simulink model "final_version"  (R2024b)
settings: Solver=FixedStepAuto  StartTime=0.0  StopTime=inf  RelTol=1e-3  EnableMultiTasking=on
libraries: simulink x46, stm32f4xxblockslib x20, dspstat3 x2, stm32blockslib x1
(part 2 of 2)

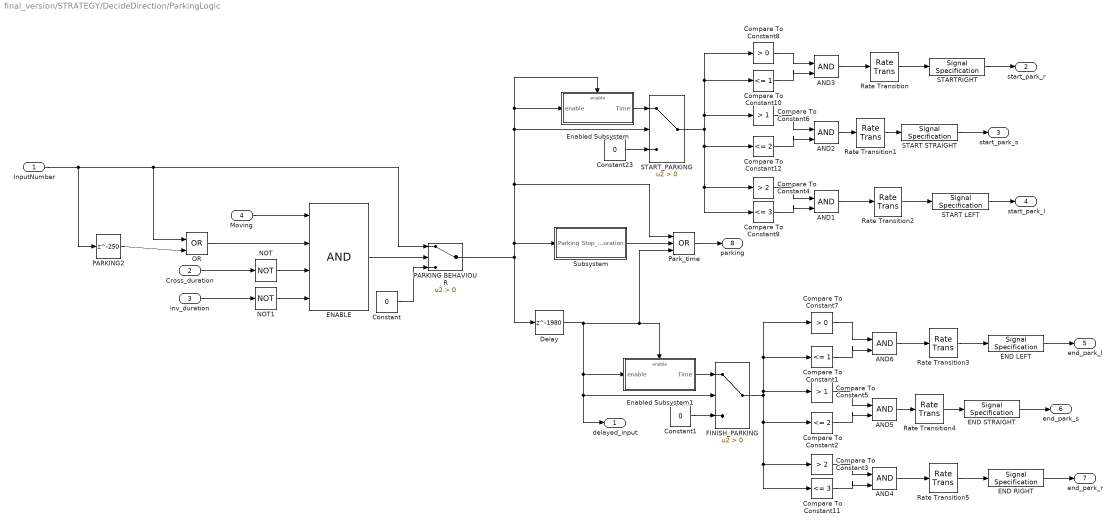
== system final_version/STRATEGY/DecideDirection/ParkingLogic ==
  InputNumber : Inport
  Cross_duration : Inport  Port=2
  inv_duration : Inport  Port=3
  Moving : Inport  Port=4
  AND{1..6} (6 alike) : Logic  IconShape=distinctive  AllPortsSameDT=off  OutDataTypeStr=boolean
  Compare To Constant1 : simulink/Logic and Bit Operations/Compare To Constant  relop=<=  const=1  OutDataTypeStr=boolean
  Compare To Constant10 : simulink/Logic and Bit Operations/Compare To Constant  relop=<=  const=1  OutDataTypeStr=boolean
  Compare To Constant11 : simulink/Logic and Bit Operations/Compare To Constant  relop=<=  const=3  OutDataTypeStr=boolean
  Compare To Constant12 : simulink/Logic and Bit Operations/Compare To Constant  relop=<=  const=2  OutDataTypeStr=boolean
  Compare To Constant2 : simulink/Logic and Bit Operations/Compare To Constant  relop=<=  const=2  OutDataTypeStr=boolean
  Compare To Constant3 : simulink/Logic and Bit Operations/Compare To Constant  relop=>  const=2  OutDataTypeStr=boolean
  Compare To Constant4 : simulink/Logic and Bit Operations/Compare To Constant  relop=>  const=2  OutDataTypeStr=boolean
  Compare To Constant5 : simulink/Logic and Bit Operations/Compare To Constant  relop=>  const=1  OutDataTypeStr=boolean
  Compare To Constant6 : simulink/Logic and Bit Operations/Compare To Constant  relop=>  const=1  OutDataTypeStr=boolean
  Compare To Constant7 : simulink/Logic and Bit Operations/Compare To Constant  relop=>  const=0  OutDataTypeStr=boolean
  Compare To Constant8 : simulink/Logic and Bit Operations/Compare To Constant  relop=>  const=0  OutDataTypeStr=boolean
  Compare To Constant9 : simulink/Logic and Bit Operations/Compare To Constant  relop=<=  const=3  OutDataTypeStr=boolean
  Constant : Constant  Value=0
  Constant1 : Constant  Value=0
  Constant23 : Constant  Value=0
  Delay : Delay  DelayLength=1980
  ENABLE : Logic  Inputs=4  IconShape=distinctive  AllPortsSameDT=off  OutDataTypeStr=boolean
  END LEFT : SignalSpecification
  END RIGHT : SignalSpecification
  END STRAIGHT : SignalSpecification
  Enabled Subsystem : Subsystem  TreatAsAtomicUnit=on
  Enabled Subsystem1 : Subsystem  TreatAsAtomicUnit=on
  FINISH_PARKING : Switch  Criteria=u2 > Threshold  SaturateOnIntegerOverflow=off  InputSameDT=off
  NOT : Logic  Operator=NOT  IconShape=distinctive  AllPortsSameDT=off  OutDataTypeStr=boolean
  NOT1 : Logic  Operator=NOT  IconShape=distinctive  AllPortsSameDT=off  OutDataTypeStr=boolean
  OR : Logic  Operator=OR  IconShape=distinctive  AllPortsSameDT=off  OutDataTypeStr=boolean
  PARKING BEHAVIOUR : Switch  Criteria=u2 > Threshold  SaturateOnIntegerOverflow=off  InputSameDT=off
  PARKING2 : Delay  DelayLength=250
  Park_time : Logic  Operator=OR  Inputs=3  IconShape=distinctive  AllPortsSameDT=off  OutDataTypeStr=boolean
  Rate Transition{,1..5} (6 alike) : RateTransition
  START LEFT : SignalSpecification
  START STRAIGHT : SignalSpecification
  STARTRIGHT : SignalSpecification
  START_PARKING : Switch  Criteria=u2 > Threshold  SaturateOnIntegerOverflow=off  InputSameDT=off
  Subsystem : Subsystem
  delayed_input : Outport
  start_park_r : Outport  Port=2
  start_park_s : Outport  Port=3
  "start_park_l " : Outport  Port=4
  end_park_l : Outport  Port=5
  end_park_s : Outport  Port=6
  end_park_r : Outport  Port=7
  parking : Outport  Port=8
  wires:
  InputNumber/1 -> PARKING BEHAVIOUR/1, OR/1, PARKING2/1
  FINISH_PARKING/1 -> Compare To Constant1/1, Compare To Constant7/1, Compare To Constant5/1, Compare To Constant2/1, Compare To Constant3/1, Compare To Constant11/1
  START_PARKING/1 -> Compare To Constant8/1, Compare To Constant10/1, Compare To Constant6/1, Compare To Constant12/1, Compare To Constant4/1, Compare To Constant9/1
  PARKING BEHAVIOUR/1 -> Delay/1, Subsystem/1(Parking), Park_time/1, START_PARKING/2, Enabled Subsystem/1(enable), Enabled Subsystem/Enable
  NOT1/1 -> ENABLE/4
  inv_duration/1 -> NOT1/1
  PARKING2/1 -> OR/2
  OR/1 -> ENABLE/2
  Moving/1 -> ENABLE/1
  NOT/1 -> ENABLE/3
  Cross_duration/1 -> NOT/1
  ENABLE/1 -> PARKING BEHAVIOUR/2
  Constant/1 -> PARKING BEHAVIOUR/3
  Compare To Constant8/1 -> AND3/1
  Compare To Constant10/1 -> AND3/2
  Compare To Constant6/1 -> AND2/1
  Compare To Constant12/1 -> AND2/2
  Compare To Constant4/1 -> AND1/1
  Compare To Constant9/1 -> AND1/2
  AND1/1 -> Rate Transition2/1
  Rate Transition2/1 -> START LEFT/1
  START LEFT/1 -> "start_park_l "/1
  START STRAIGHT/1 -> start_park_s/1
  STARTRIGHT/1 -> start_park_r/1
  Rate Transition/1 -> STARTRIGHT/1
  Rate Transition1/1 -> START STRAIGHT/1
  AND2/1 -> Rate Transition1/1
  AND3/1 -> Rate Transition/1
  Constant23/1 -> START_PARKING/3
  Enabled Subsystem/1(Time) -> START_PARKING/1
  Delay/1 -> Park_time/3, Enabled Subsystem1/Enable, Enabled Subsystem1/1(enable), delayed_input/1, FINISH_PARKING/2
  Park_time/1 -> parking/1
  Subsystem/1(Stop_duration) -> Park_time/2
  Constant1/1 -> FINISH_PARKING/3
  Enabled Subsystem1/1(Time) -> FINISH_PARKING/1
  Compare To Constant1/1 -> AND6/2
  Compare To Constant7/1 -> AND6/1
  Compare To Constant5/1 -> AND5/1
  Compare To Constant2/1 -> AND5/2
  Compare To Constant3/1 -> AND4/1
  Compare To Constant11/1 -> AND4/2
  AND4/1 -> Rate Transition5/1
  Rate Transition5/1 -> END RIGHT/1
  END RIGHT/1 -> end_park_r/1
  END STRAIGHT/1 -> end_park_s/1
  END LEFT/1 -> end_park_l/1
  Rate Transition3/1 -> END LEFT/1
  Rate Transition4/1 -> END STRAIGHT/1
  AND5/1 -> Rate Transition4/1
  AND6/1 -> Rate Transition3/1

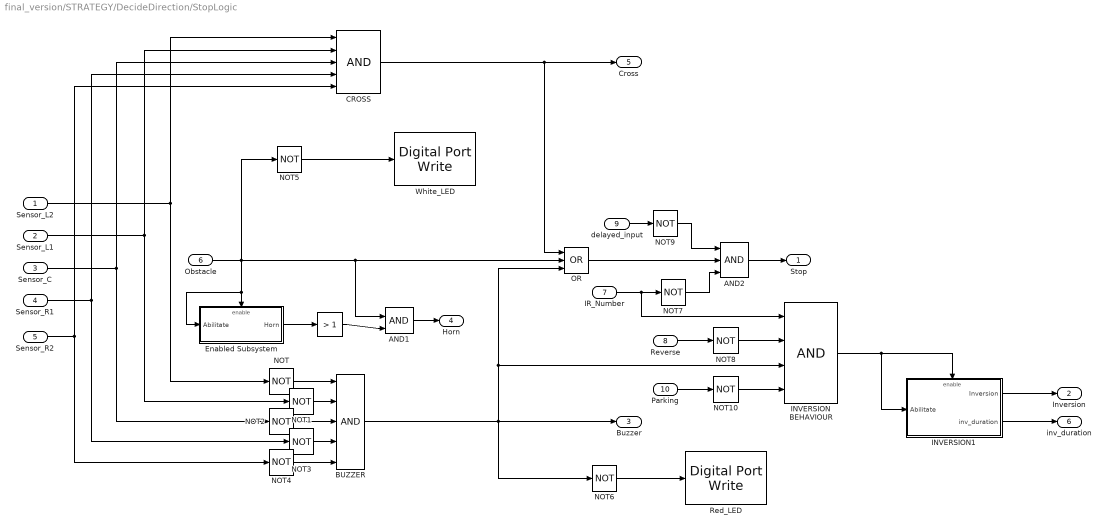
== system final_version/STRATEGY/DecideDirection/StopLogic ==
  Sensor_L2 : Inport
  Sensor_L1 : Inport  Port=2
  Sensor_C : Inport  Port=3
  Sensor_R1 : Inport  Port=4
  Sensor_R2 : Inport  Port=5
  Obstacle : Inport  Port=6
  IR_Number : Inport  Port=7
  Reverse : Inport  Port=8
  delayed_input : Inport  Port=9
  Parking : Inport  Port=10
  " " : simulink/Logic and Bit Operations/Compare To Constant  relop=>  const=1  OutDataTypeStr=boolean
  AND1 : Logic  IconShape=distinctive  AllPortsSameDT=off  OutDataTypeStr=boolean
  AND2 : Logic  Inputs=3  IconShape=distinctive  AllPortsSameDT=off  OutDataTypeStr=boolean
  BUZZER : Logic  Inputs=5  IconShape=distinctive  AllPortsSameDT=off  OutDataTypeStr=boolean
  CROSS : Logic  Inputs=5  IconShape=distinctive  AllPortsSameDT=off  OutDataTypeStr=boolean
  Enabled Subsystem : Subsystem  TreatAsAtomicUnit=on
  INVERSION BEHAVIOUR : Logic  Inputs=4  IconShape=distinctive  AllPortsSameDT=off  OutDataTypeStr=boolean
  INVERSION1 : Subsystem  TreatAsAtomicUnit=on
  NOT{,1..10} (11 alike) : Logic  Operator=NOT  IconShape=distinctive  AllPortsSameDT=off  OutDataTypeStr=boolean
  OR : Logic  Operator=OR  Inputs=3  IconShape=distinctive  AllPortsSameDT=off  OutDataTypeStr=boolean
  Red_LED : stm32f4xxblockslib/Digital Port Write  PortName=GPIOC  PinNumber=[6]  ReadOperation=off  IOAsArray=on  EnableSimPort=off  hoistedMaskSrc=ECSoC/ECSimCodegen/Digital Port Write
  White_LED : stm32f4xxblockslib/Digital Port Write  PortName=GPIOC  PinNumber=[9]  ReadOperation=off  IOAsArray=on  EnableSimPort=off  hoistedMaskSrc=ECSoC/ECSimCodegen/Digital Port Write
  Stop : Outport
  Inversion : Outport  Port=2
  Buzzer : Outport  Port=3
  Horn : Outport  Port=4
  Cross : Outport  Port=5
  inv_duration : Outport  Port=6
  wires:
  Sensor_L2/1 -> NOT/1, CROSS/1
  Sensor_L1/1 -> CROSS/2, NOT1/1
  Sensor_C/1 -> CROSS/3, NOT2/1
  Sensor_R1/1 -> CROSS/4, NOT3/1
  Sensor_R2/1 -> CROSS/5, NOT4/1
  CROSS/1 -> Cross/1, OR/1
  NOT/1 -> BUZZER/1
  NOT1/1 -> BUZZER/2
  NOT2/1 -> BUZZER/3
  NOT3/1 -> BUZZER/4
  NOT4/1 -> BUZZER/5
  Obstacle/1 -> NOT5/1, AND1/1, OR/2, Enabled Subsystem/1(Abilitate), Enabled Subsystem/Enable
  Enabled Subsystem/1(Horn) -> " "/1
  NOT5/1 -> White_LED/1
  NOT6/1 -> Red_LED/1
  INVERSION1/1(Inversion) -> Inversion/1
  AND2/1 -> Stop/1
  IR_Number/1 -> NOT7/1, INVERSION BEHAVIOUR/1
  AND1/1 -> Horn/1
  " "/1 -> AND1/2
  Reverse/1 -> NOT8/1
  BUZZER/1 -> NOT6/1, OR/3, INVERSION BEHAVIOUR/3, Buzzer/1
  NOT7/1 -> AND2/3
  OR/1 -> AND2/2
  delayed_input/1 -> NOT9/1
  NOT9/1 -> AND2/1
  NOT8/1 -> INVERSION BEHAVIOUR/2
  Parking/1 -> NOT10/1
  NOT10/1 -> INVERSION BEHAVIOUR/4
  INVERSION BEHAVIOUR/1 -> INVERSION1/1(Abilitate), INVERSION1/Enable
  INVERSION1/2(inv_duration) -> inv_duration/1

== system final_version/STRATEGY/DecideDirection/TurnLeftLogic ==
  Sensor_L2 : Inport
  Sensor_L1 : Inport  Port=2
  Sensor_C : Inport  Port=3
  Inversion : Inport  Port=4
  cross_duration : Inport  Port=5
  start_park_r : Inport  Port=6
  end_park_r : Inport  Port=7
  AND : Logic  IconShape=distinctive  AllPortsSameDT=off  OutDataTypeStr=boolean
  AND1 : Logic  Inputs=3  IconShape=distinctive  AllPortsSameDT=off  OutDataTypeStr=boolean
  AND2 : Logic  Inputs=5  IconShape=distinctive  AllPortsSameDT=off  OutDataTypeStr=boolean
  NOT{1..5} (5 alike) : Logic  Operator=NOT  IconShape=distinctive  AllPortsSameDT=off  OutDataTypeStr=boolean
  OR : Logic  Operator=OR  IconShape=distinctive  AllPortsSameDT=off  OutDataTypeStr=boolean
  Turn_Left : Outport
  wires:
  NOT3/1 -> AND/2
  AND/1 -> OR/1
  Sensor_L1/1 -> NOT3/1, AND1/1
  Sensor_L2/1 -> AND1/2, AND/1
  Sensor_C/1 -> AND1/3
  AND1/1 -> OR/2
  Inversion/1 -> NOT1/1
  OR/1 -> AND2/1
  NOT1/1 -> AND2/2
  AND2/1 -> Turn_Left/1
  NOT2/1 -> AND2/3
  cross_duration/1 -> NOT2/1
  start_park_r/1 -> NOT4/1
  NOT4/1 -> AND2/4
  end_park_r/1 -> NOT5/1
  NOT5/1 -> AND2/5

== system final_version/STRATEGY/DecideDirection/TurnRightLogic ==
  Sensor_R2 : Inport
  Sensor_R1 : Inport  Port=2
  Sensor_C : Inport  Port=3
  inversion : Inport  Port=4
  cross_duration : Inport  Port=5
  start_park_r : Inport  Port=6
  end_park_r : Inport  Port=7
  AND : Logic  Inputs=3  IconShape=distinctive  AllPortsSameDT=off  OutDataTypeStr=boolean
  AND1 : Logic  IconShape=distinctive  AllPortsSameDT=off  OutDataTypeStr=boolean
  AND2 : Logic  Inputs=4  IconShape=distinctive  AllPortsSameDT=off  OutDataTypeStr=boolean
  NOT{1..4} (4 alike) : Logic  Operator=NOT  IconShape=distinctive  AllPortsSameDT=off  OutDataTypeStr=boolean
  OR1 : Logic  Operator=OR  IconShape=distinctive  AllPortsSameDT=off  OutDataTypeStr=boolean
  XOR : Logic  Operator=XOR  IconShape=distinctive  AllPortsSameDT=off  OutDataTypeStr=boolean
  Turn_Right : Outport
  wires:
  AND1/1 -> OR1/1
  NOT4/1 -> AND1/2
  Sensor_R1/1 -> AND/1, NOT4/1
  Sensor_R2/1 -> AND/2, AND1/1
  inversion/1 -> XOR/2
  AND/1 -> OR1/2
  Sensor_C/1 -> AND/3
  AND2/1 -> Turn_Right/1
  NOT1/1 -> AND2/2
  cross_duration/1 -> NOT1/1
  start_park_r/1 -> NOT2/1
  NOT2/1 -> AND2/3
  end_park_r/1 -> NOT3/1
  NOT3/1 -> AND2/4
  XOR/1 -> AND2/1
  OR1/1 -> XOR/1

== system final_version/STRATEGY/DecideDirection/TurnSlightLeftLogic ==
  Sensor_C : Inport
  Sensor_L1 : Inport  Port=2
  Sensor_L2 : Inport  Port=3
  start_park_l : Inport  Port=4
  end_park_l : Inport  Port=5
  start_park_r : Inport  Port=6
  end_park_r : Inport  Port=7
  Inversion : Inport  Port=8
  x_left : Inport  Port=9
  AND : Logic  Inputs=3  IconShape=distinctive  AllPortsSameDT=off  OutDataTypeStr=boolean
  AND1 : Logic  Inputs=4  IconShape=distinctive  AllPortsSameDT=off  OutDataTypeStr=boolean
  NOT{,1..3} (4 alike) : Logic  Operator=NOT  IconShape=distinctive  AllPortsSameDT=off  OutDataTypeStr=boolean
  OR : Logic  Operator=OR  Inputs=4  IconShape=distinctive  AllPortsSameDT=off  OutDataTypeStr=boolean
  TurnSlightLeft : Outport
  wires:
  Sensor_C/1 -> NOT/1
  Sensor_L1/1 -> AND/2
  NOT/1 -> AND/1
  AND/1 -> OR/1
  end_park_l/1 -> OR/3
  AND1/1 -> TurnSlightLeft/1
  OR/1 -> AND1/1
  NOT1/1 -> AND1/2
  start_park_r/1 -> NOT1/1
  start_park_l/1 -> OR/2
  Sensor_L2/1 -> AND/3
  Inversion/1 -> NOT2/1
  NOT2/1 -> AND1/3
  x_left/1 -> OR/4
  end_park_r/1 -> NOT3/1
  NOT3/1 -> AND1/4

== system final_version/STRATEGY/DecideDirection/TurnSlightRightLogic ==
  Sensor_R1 : Inport
  Sensor_R2 : Inport  Port=2
  Sensor_C : Inport  Port=3
  start_park_r : Inport  Port=4
  end_park_r : Inport  Port=5
  Inversion : Inport  Port=6
  x_right : Inport  Port=7
  AND : Logic  Inputs=3  IconShape=distinctive  AllPortsSameDT=off  OutDataTypeStr=boolean
  AND1 : Logic  IconShape=distinctive  AllPortsSameDT=off  OutDataTypeStr=boolean
  NOT1 : Logic  Operator=NOT  IconShape=distinctive  AllPortsSameDT=off  OutDataTypeStr=boolean
  NOT2 : Logic  Operator=NOT  IconShape=distinctive  AllPortsSameDT=off  OutDataTypeStr=boolean
  OR : Logic  Operator=OR  Inputs=4  IconShape=distinctive  AllPortsSameDT=off  OutDataTypeStr=boolean
  TurnSlightRight : Outport
  wires:
  Sensor_C/1 -> NOT2/1
  Sensor_R1/1 -> AND/1
  AND/1 -> OR/1
  end_park_r/1 -> OR/3
  start_park_r/1 -> OR/2
  NOT2/1 -> AND/3
  Sensor_R2/1 -> AND/2
  AND1/1 -> TurnSlightRight/1
  OR/1 -> AND1/1
  Inversion/1 -> NOT1/1
  NOT1/1 -> AND1/2
  x_right/1 -> OR/4

== system final_version/STRATEGY/DecideDirection/UltrasonicLogic ==
  UT : Inport
  Clock : Clock
  Clock1 : Clock
  Constant : Constant  Value=11.7
  Constant1 : Constant  Value=9.3
  OBSTACLE : RelationalOperator  Operator=<  OutDataTypeStr=boolean  RndMeth=Simplest  InputSameDT=off
  REVERSE : RelationalOperator  Operator=<  OutDataTypeStr=boolean  RndMeth=Simplest  InputSameDT=off
  obstacle : Logic  IconShape=distinctive  AllPortsSameDT=off  OutDataTypeStr=boolean
  obstacle clock : simulink/Logic and Bit Operations/Compare To Constant  relop=>=  const=0.25  OutDataTypeStr=boolean
  reverse : Logic  IconShape=distinctive  AllPortsSameDT=off  OutDataTypeStr=boolean
  reverse clock : simulink/Logic and Bit Operations/Compare To Constant  relop=>=  const=0.25  OutDataTypeStr=boolean
  Obstacle : Outport
  Reverse : Outport  Port=2
  wires:
  Clock1/1 -> reverse clock/1
  Constant1/1 -> REVERSE/2
  Clock/1 -> obstacle clock/1
  reverse clock/1 -> reverse/2
  Constant/1 -> OBSTACLE/2
  UT/1 -> OBSTACLE/1, REVERSE/1
  obstacle clock/1 -> obstacle/1
  OBSTACLE/1 -> obstacle/2
  reverse/1 -> Reverse/1
  obstacle/1 -> Obstacle/1
  REVERSE/1 -> reverse/1

== system final_version/STRATEGY/Forward_LED_routine/Enabled Subsystem ==
  Enable : EnablePort  StatesWhenEnabling=reset
  Constant1 : Constant  Value=4
  Data Type Conversion1 : DataTypeConversion  OutDataTypeStr=uint16  SaturateOnIntegerOverflow=off  RndMeth=Floor
  Mod : Math  Operator=rem
  Pulse Generator1 : DiscretePulseGenerator  PulseType=Time based  Period=0.1  PulseWidth=50
  Relational Operator1 : RelationalOperator  Operator=>  OutDataTypeStr=boolean  RndMeth=Simplest  InputSameDT=off
  Sum : Sum
  Unit Delay : UnitDelay  SampleTime=-1  HasFrameUpgradeWarning=on
  Unit Delay1 : UnitDelay  SampleTime=-1  HasFrameUpgradeWarning=on
  LED_selector : Outport
  wires:
  Mod/1 -> LED_selector/1
  Constant1/1 -> Mod/2
  Unit Delay/1 -> Relational Operator1/2
  Relational Operator1/1 -> Data Type Conversion1/1
  Unit Delay1/1 -> Sum/2
  Data Type Conversion1/1 -> Sum/1
  Sum/1 -> Mod/1, Unit Delay1/1
  Pulse Generator1/1 -> Unit Delay/1, Relational Operator1/1

== system final_version/STRATEGY/DecideDirection/ParkingLogic/Enabled Subsystem ==
  enable : Inport
  Enable : EnablePort  StatesWhenEnabling=reset
  Constant : Constant  Value=0
  Data Type Conversion : DataTypeConversion  OutDataTypeStr=uint16  SaturateOnIntegerOverflow=off  RndMeth=Floor
  Pulse Generator : DiscretePulseGenerator  PulseType=Time based  Period=0.065  PulseWidth=50
  Relational Operator : RelationalOperator  Operator=>  OutDataTypeStr=boolean  RndMeth=Simplest  InputSameDT=off
  Sum : Sum
  Switch : Switch  Criteria=u2 > Threshold  SaturateOnIntegerOverflow=off  InputSameDT=off
  Unit Delay : UnitDelay  SampleTime=-1  HasFrameUpgradeWarning=on
  Unit Delay1 : UnitDelay  SampleTime=-1  HasFrameUpgradeWarning=on
  Time : Outport
  wires:
  Unit Delay/1 -> Relational Operator/2
  Relational Operator/1 -> Data Type Conversion/1
  Unit Delay1/1 -> Sum/2
  Sum/1 -> Unit Delay1/1, Time/1
  Data Type Conversion/1 -> Sum/1
  Pulse Generator/1 -> Switch/1
  enable/1 -> Switch/2
  Constant/1 -> Switch/3
  Switch/1 -> Unit Delay/1, Relational Operator/1

== system final_version/STRATEGY/DecideDirection/ParkingLogic/Enabled Subsystem1 ==
  enable : Inport
  Enable : EnablePort  StatesWhenEnabling=reset
  Constant : Constant  Value=0
  Data Type Conversion : DataTypeConversion  OutDataTypeStr=uint16  SaturateOnIntegerOverflow=off  RndMeth=Floor
  Pulse Generator : DiscretePulseGenerator  PulseType=Time based  Period=.07  PulseWidth=50
  Relational Operator : RelationalOperator  Operator=>  OutDataTypeStr=boolean  RndMeth=Simplest  InputSameDT=off
  Sum : Sum
  Switch : Switch  Criteria=u2 > Threshold  SaturateOnIntegerOverflow=off  InputSameDT=off
  Unit Delay : UnitDelay  SampleTime=-1  HasFrameUpgradeWarning=on
  Unit Delay1 : UnitDelay  SampleTime=-1  HasFrameUpgradeWarning=on
  Time : Outport
  wires:
  Unit Delay/1 -> Relational Operator/2
  Relational Operator/1 -> Data Type Conversion/1
  Unit Delay1/1 -> Sum/2
  Sum/1 -> Time/1, Unit Delay1/1
  Data Type Conversion/1 -> Sum/1
  enable/1 -> Switch/2
  Constant/1 -> Switch/3
  Pulse Generator/1 -> Switch/1
  Switch/1 -> Relational Operator/1, Unit Delay/1

== system final_version/STRATEGY/DecideDirection/ParkingLogic/Subsystem ==
  Parking : Inport
  Delay : Delay  DelayLength=304
  Delay1 : Delay  DelayLength=2*304
  Delay2 : Delay  DelayLength=4*304
  Delay3 : Delay  DelayLength=304*5
  Delay4 : Delay  DelayLength=304*6
  Delay6 : Delay  DelayLength=3*304
  OR : Logic  Operator=OR  Inputs=6  IconShape=distinctive  AllPortsSameDT=off  OutDataTypeStr=boolean
  Stop_duration : Outport
  wires:
  Parking/1 -> Delay6/1, Delay1/1, Delay/1, Delay2/1, Delay4/1, Delay3/1
  OR/1 -> Stop_duration/1
  Delay/1 -> OR/1
  Delay1/1 -> OR/2
  Delay6/1 -> OR/3
  Delay2/1 -> OR/4
  Delay3/1 -> OR/5
  Delay4/1 -> OR/6

== system final_version/STRATEGY/DecideDirection/StopLogic/Enabled Subsystem ==
  Abilitate : Inport
  Distance_UT : EnablePort  StatesWhenEnabling=reset
  Constant1 : Constant  Value=0
  Data Type Conversion : DataTypeConversion  OutDataTypeStr=uint16  SaturateOnIntegerOverflow=off  RndMeth=Floor
  Pulse Generator : DiscretePulseGenerator  PulseType=Time based  Period=0.2  PulseWidth=50
  Relational Operator : RelationalOperator  Operator=>  OutDataTypeStr=boolean  RndMeth=Simplest  InputSameDT=off
  Sum : Sum
  Switch : Switch  Criteria=u2 > Threshold  SaturateOnIntegerOverflow=off  InputSameDT=off
  Unit Delay : UnitDelay  SampleTime=-1  HasFrameUpgradeWarning=on
  Unit Delay1 : UnitDelay  SampleTime=-1  HasFrameUpgradeWarning=on
  Horn : Outport
  wires:
  Unit Delay1/1 -> Sum/2
  Unit Delay/1 -> Relational Operator/2
  Data Type Conversion/1 -> Sum/1
  Sum/1 -> Horn/1, Unit Delay1/1
  Relational Operator/1 -> Data Type Conversion/1
  Switch/1 -> Unit Delay/1, Relational Operator/1
  Abilitate/1 -> Switch/2
  Pulse Generator/1 -> Switch/1
  Constant1/1 -> Switch/3

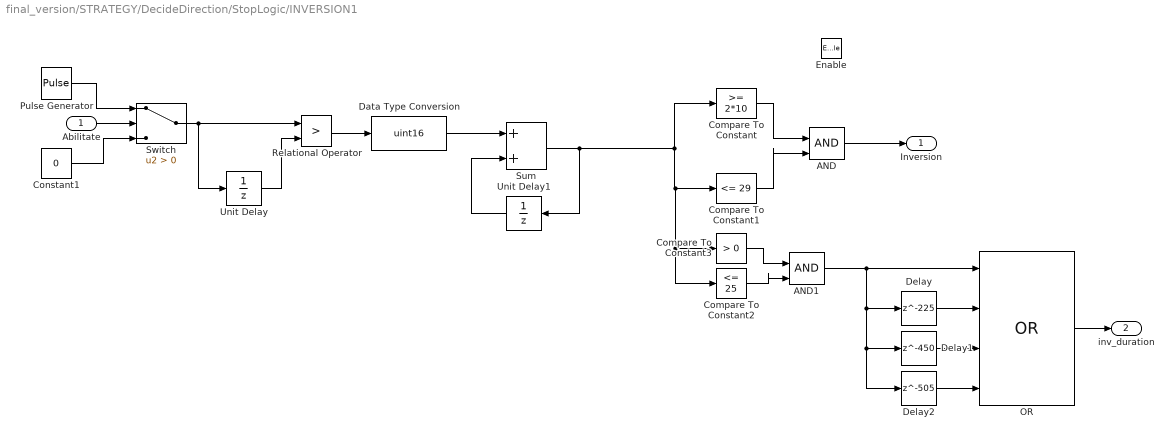
== system final_version/STRATEGY/DecideDirection/StopLogic/INVERSION1 ==
  Abilitate : Inport
  Enable : EnablePort  StatesWhenEnabling=reset
  AND : Logic  IconShape=distinctive  AllPortsSameDT=off  OutDataTypeStr=boolean
  AND1 : Logic  IconShape=distinctive  AllPortsSameDT=off  OutDataTypeStr=boolean
  Compare To Constant : simulink/Logic and Bit Operations/Compare To Constant  relop=>=  const=2*10  OutDataTypeStr=boolean
  Compare To Constant1 : simulink/Logic and Bit Operations/Compare To Constant  relop=<=  const=29  OutDataTypeStr=boolean
  Compare To Constant2 : simulink/Logic and Bit Operations/Compare To Constant  relop=<=  const=25  OutDataTypeStr=boolean
  Compare To Constant3 : simulink/Logic and Bit Operations/Compare To Constant  relop=>  const=0  OutDataTypeStr=boolean
  Constant1 : Constant  Value=0
  Data Type Conversion : DataTypeConversion  OutDataTypeStr=uint16  SaturateOnIntegerOverflow=off  RndMeth=Floor
  Delay : Delay  DelayLength=225
  Delay1 : Delay  DelayLength=450
  Delay2 : Delay  DelayLength=505
  OR : Logic  Operator=OR  Inputs=4  IconShape=distinctive  AllPortsSameDT=off  OutDataTypeStr=boolean
  Pulse Generator : DiscretePulseGenerator  PulseType=Time based  Period=0.1/10  PulseWidth=50
  Relational Operator : RelationalOperator  Operator=>  OutDataTypeStr=boolean  RndMeth=Simplest  InputSameDT=off
  Sum : Sum
  Switch : Switch  Criteria=u2 > Threshold  SaturateOnIntegerOverflow=off  InputSameDT=off
  Unit Delay : UnitDelay  SampleTime=-1  HasFrameUpgradeWarning=on
  Unit Delay1 : UnitDelay  SampleTime=-1  HasFrameUpgradeWarning=on
  Inversion : Outport
  inv_duration : Outport  Port=2
  wires:
  Compare To Constant/1 -> AND/1
  Compare To Constant1/1 -> AND/2
  AND/1 -> Inversion/1
  Unit Delay1/1 -> Sum/2
  Unit Delay/1 -> Relational Operator/2
  Data Type Conversion/1 -> Sum/1
  Relational Operator/1 -> Data Type Conversion/1
  Switch/1 -> Unit Delay/1, Relational Operator/1
  Pulse Generator/1 -> Switch/1
  Constant1/1 -> Switch/3
  Abilitate/1 -> Switch/2
  Sum/1 -> Compare To Constant/1, Compare To Constant2/1, Compare To Constant3/1, Compare To Constant1/1, Unit Delay1/1
  Delay/1 -> OR/2
  OR/1 -> inv_duration/1
  Compare To Constant2/1 -> AND1/2
  Compare To Constant3/1 -> AND1/1
  AND1/1 -> OR/1, Delay/1, Delay1/1, Delay2/1
  Delay2/1 -> OR/4
  Delay1/1 -> OR/3

== matlab function final_version/STM32 Nucleo F411RE INPUT/IR_remote_logic/resetted_max ==
  data: x input; y output
function y = resetted_max(x)
    % Declare the persistent variable
    persistent max_value zero_count reset_flag;
    sample_time = 1;

    % Define the zero threshold 
    zero_threshold_time = 5; % seconds
    zero_threshold_samples = round(zero_threshold_time / sample_time);

    % Initailize the persistent variable
    if isempty(max_value)
        max_value = -inf;     % Initialize the maximum 
        zero_count = 0;       % Counter of zero samples
        reset_flag = false;   % Resetted max flag
    end

    % If signal is zero increase the counter 
    if x == 0
        zero_count = zero_count + 1;
        
        % If the signal is zero for long enough reset the signal
        if zero_count >= zero_threshold_samples
            max_value = -inf;  % Maximum reset
            reset_flag = true; 
        end
        
    else
        % If signal is different from zero reset the counter and adjust the maximum
        zero_count = 0; 
        
        if reset_flag
            % If we were in reset phase reset and strat from zero to search for the maximum
            max_value = x;     
            reset_flag = false;
        else
            % Update the maixmum if not in reset phase
            max_value = max(max_value, x);
        end
    end

    % If the signal was zero for 5 seconds return zero otherwise the maximum
    if zero_count >= zero_threshold_samples
        y = 0;
    else
        y = max_value;
    end
end

== matlab function final_version/STRATEGY/CalculatePins/MATLAB Function - Calculate Pins ==
  data: f input; rp1 output; tr input; tl input; tsr input; tsl input; s input; rev input; rp2 output; lp1 output; lp2 output; spr output; spl output; speed input; isturning output
function [rp1,rp2,lp1,lp2,spr,spl,isturning] = fcn(f,tr,tl,tsr,tsl,s,rev,speed)
    rp1 = 0;
    rp2 = 0;
    lp1 = 0;
    lp2 = 0;
    spr = 0;
    spl = 0;
    isturning = false;
if f % Forward pin setup
    rp1 = 0;
    rp2 = 1;
    lp1 = 0;
    lp2 = 1;
    spr = speed;
    spl = speed;
    isturning = false;
end
if tr % Turn Right pin setup
    rp1 = 1;
    rp2 = 0;
    lp1 = 0;
    lp2 = 1;
    spr = speed;
    spl = speed;
    isturning = true;
end
if tl % Turn Left pin setup
    rp1 = 0;
    rp2 = 1;
    lp1 = 1;
    lp2 = 0;
    spr = speed;
    spl = speed;
    isturning = true;
end
if tsr % Turn Slight Right pin setup
    rp1 = 0;
    rp2 = 1;
    lp1 = 0;
    lp2 = 1;
    spr = 0;
    spl = speed;
    isturning = true;
end
if tsl % Turn Slight Left pin setup
    rp1 = 0;
    rp2 = 1;
    lp1 = 0;
    lp2 = 1;
    spr = speed;
    spl = 0;
    isturning = true;
end
if s % Stop pin setup
    rp1 = 0;
    rp2 = 0;
    lp1 = 0;
    lp2 = 0;
    spr = 0;
    spl = 0;
    isturning = false;
end
if rev % Reverse pin setup
    rp1 = 1;
    rp2 = 0;
    lp1 = 1;
    lp2 = 0;
    spr = speed;
    spl = speed;
    isturning = false;    
end
end
